simulink library "VISMODAL_MASTER"  (Simulink 8.6)
settings: Solver=VariableStepAuto  StartTime=0.0  StopTime=10.0  RelTol=1e-3
libraries: VIS_LIB x140, cdsFilt x34, cdsMuxMatrix x6, VISMODAL_MASTER x1
(part 1 of 5)
settings Model: Creator=controls  LastModifiedBy=controls

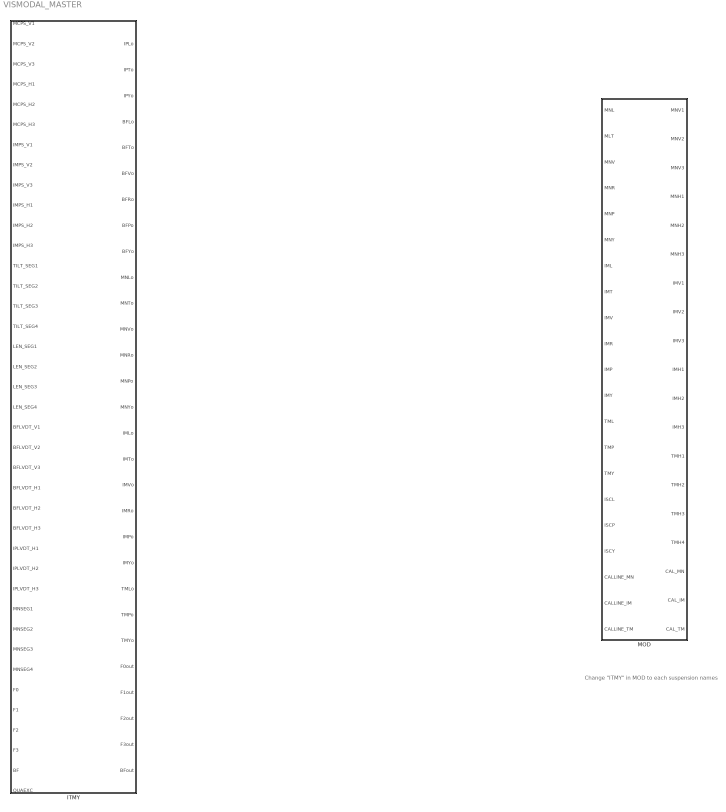
== system VISMODAL_MASTER ==
  note: Change "ITMY" in MOD to each suspension names
  ITMY : Subsystem
  MOD : Subsystem  Tag=top_names
